simulink model "Vector_projection_get_closest_point"  (R2021a)
settings: configuration reference "AION_IDS_Speedgoat" (kept outside this file)
libraries: simulink x1
Description:
  | 向量投影法获取线段P1P2上距离当前点P的最近点C
settings Model: DataDictionary=Vector_Projection_Get_Closest_Point.sldd  Creator=xinrui  LastModifiedBy=Administrator
settings ConfigSetRef: SourceName=AION_IDS_Speedgoat

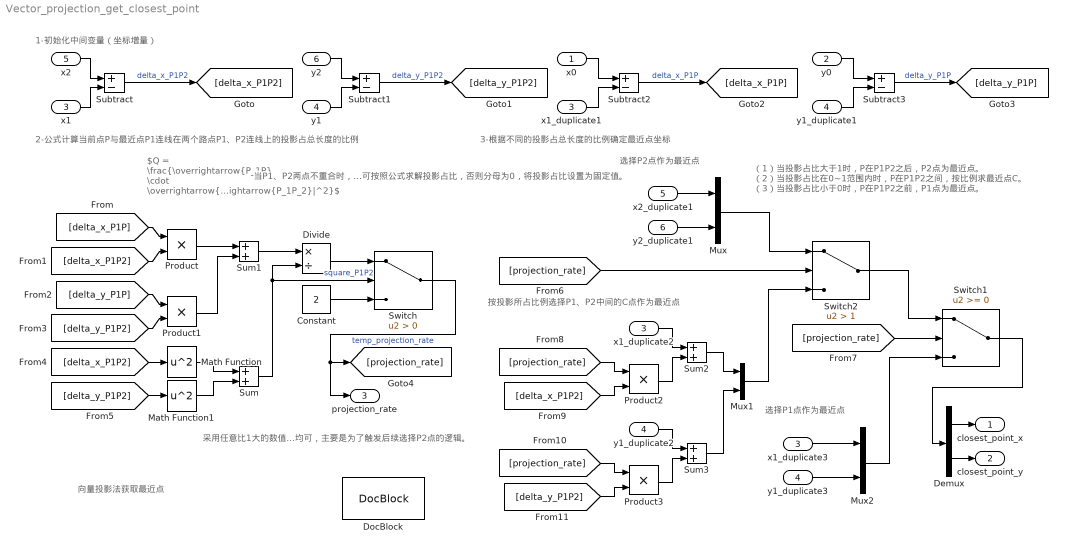
== system Vector_projection_get_closest_point ==
  note: $Q = \frac{\overrightarrow{P_1P} \cdot \overrightarrow{P_1P_2}}{|\overrightarrow{P_1P_2}|^2}$
  note: 当P1、P2两点不重合时，可按照公式求解投影占比，否则分母为0，将投影占比设置为固定值。
  note: （1）当投影占比大于1时，P在P1P2之后，P2点为最近点。
      | （2）当投影占比在0~1范围内时，P在P1P2之间，按比例求最近点C。
      | （3）当投影占比小于0时，P在P1P2之前，P1点为最近点。
  note: 向量投影法获取最近点
  note: 选择P1点作为最近点
  note: 按投影所占比例选择P1、P2中间的C点作为最近点
  note: 选择P2点作为最近点
  note: 采用任意比1大的数值均可，主要是为了触发后续选择P2点的逻辑。
  note: 3-根据不同的投影占总长度的比例确定最近点坐标
  note: 2-公式计算当前点P与最近点P1连线在两个路点P1、P2连线上的投影占总长度的比例
  note: 1-初始化中间变量（坐标增量）
  x0 : Inport  Description=当前点P的x坐标，实数，m。  OutDataTypeStr=double  PortDimensions=1
  y0 : Inport  Description=当前点P的y坐标，实数，m。  Port=2  OutDataTypeStr=double  PortDimensions=1
  x1 : Inport  Description=路点线段起始端点P1的x坐标，实数，m。  Port=3  OutDataTypeStr=double  PortDimensions=1
  y1 : Inport  Description=路点线段起始端点P1的y坐标，实数，m。  Port=4  OutDataTypeStr=double  PortDimensions=1
  x2 : Inport  Description=路点线段终止端点P2的x坐标，实数，m。  Port=5  OutDataTypeStr=double  PortDimensions=1
  y2 : Inport  Description=路点线段终止端点P2的y坐标，实数，m。  Port=6  OutDataTypeStr=double  PortDimensions=1
  Constant : Constant  Description=采用任意比1大的数值均可，主要是为了触发后续选择P2点的逻辑。  Value=2  OutDataTypeStr=double
  Demux : Demux  Outputs=2
  Divide : Product  Description=公式计算当前点P与最近点P1连线在两个路点P1、P2连线上的投影占总长度的比例  Inputs=*/
  DocBlock : simulink/Model-Wide Utilities/DocBlock  DocumentType=HTML  mask(DocBlock){}
      mask Display:
      | plot([.8 0 0 1 1 .8 .8 1],[1 1 0 0 .8 1 .8 .8]);
      | text(.5,.6,'CHANGELOG','horizontalalignment','center');
      | text(.95,.05,get_param(gcb,'DocumentType'),'verticalalignment','bottom','horizontalalignment','right');
  Math Function : Math  Operator=square  SaturateOnIntegerOverflow=on
  Math Function1 : Math  Operator=square  SaturateOnIntegerOverflow=on
  Mux : Mux  Inputs=2
  Mux1 : Mux  Inputs=2
  Mux2 : Mux  Inputs=2
  Product{,1..3} (4 alike) : Product
  Subtract : Sum  Description=计算线段P1P2的x坐标增量。  Inputs=+-
  Subtract1 : Sum  Description=计算线段P1P2的y坐标增量。  Inputs=+-
  Subtract2 : Sum  Description=计算线段P1P的x坐标增量。  Inputs=+-
  Subtract3 : Sum  Description=计算线段P1P的y坐标增量。  Inputs=+-
  Sum : Sum  Description=计算线段P1P2的距离平方，以判断公式分母是否为零。
  Sum1 : Sum
  Sum2 : Sum  Description=按投影所占比例选择P1、P2中间的C点作为最近点。
  Sum3 : Sum  Description=按投影所占比例选择P1、P2中间的C点作为最近点。
  Switch : Switch  Description=当P1、P2两点不重合时，可按照公式求解投影占比，否则分母为0，将投影占比设置为固定值。  Criteria=u2 > Threshold  OutDataTypeStr=double
  Switch1 : Switch  Description=|  OutDataTypeStr=double
      | （1）当投影占比大于1时，P在P1P2之后，P2点为最近点。
      | （2）当投影占比在0~1范围内时，P在P1P2之间，按比例求最近点C。
      | （3）当投影占比小于0时，P在P1P2之前，P1点为最近点。
  Switch2 : Switch  Description=|  Criteria=u2 > Threshold  Threshold=1  OutDataTypeStr=double
      | （1）当投影占比大于1时，P在P1P2之后，P2点为最近点。
      | （2）当投影占比在0~1范围内时，P在P1P2之间，按比例求最近点C。
      | （3）当投影占比小于0时，P在P1P2之前，P1点为最近点。
  x1_duplicate1 : InportShadow  Port=3  OutDataTypeStr=double  PortDimensions=1
  x1_duplicate2 : InportShadow  Port=3  OutDataTypeStr=double  PortDimensions=1
  x1_duplicate3 : InportShadow  Port=3  OutDataTypeStr=double  PortDimensions=1
  x2_duplicate1 : InportShadow  Port=5  OutDataTypeStr=double  PortDimensions=1
  y1_duplicate1 : InportShadow  Port=4  OutDataTypeStr=double  PortDimensions=1
  y1_duplicate2 : InportShadow  Port=4  OutDataTypeStr=double  PortDimensions=1
  y1_duplicate3 : InportShadow  Port=4  OutDataTypeStr=double  PortDimensions=1
  y2_duplicate1 : InportShadow  Port=6  OutDataTypeStr=double  PortDimensions=1
  closest_point_x : Outport  Description=路点线段上距离当前点P最近的点C的x坐标，实数，m。  OutDataTypeStr=double  PortDimensions=1
  closest_point_y : Outport  Description=路点线段上距离当前点P最近的点C的y坐标，实数，m。  Port=2  OutDataTypeStr=double  PortDimensions=1
  projection_rate : Outport  Description=当前点P与线段起始点P1连线在两个路点P1、P2连线上的投影占总长度的比例，实数，无量纲。  Port=3  OutDataTypeStr=double  PortDimensions=1
  wires:
  x0/1 -> Subtract2/1
  x2/1 -> Subtract/1
  x1/1 -> Subtract/2
  y2/1 -> Subtract1/1
  y1/1 -> Subtract1/2
  y0/1 -> Subtract3/1
  Math Function/1 -> Sum/1
  Math Function1/1 -> Sum/2
  Sum/1 -> Divide/2, Switch/2  "square_P1P2"
  Product/1 -> Sum1/1
  Product1/1 -> Sum1/2
  Sum1/1 -> Divide/1
  Divide/1 -> Switch/1
  Constant/1 -> Switch/3
  Mux/1 -> Switch2/1
  Product2/1 -> Sum2/2
  Product3/1 -> Sum3/2
  Sum2/1 -> Mux1/1
  Sum3/1 -> Mux1/2
  Mux1/1 -> Switch2/3
  Switch2/1 -> Switch1/1
  Mux2/1 -> Switch1/3
  Switch1/1 -> Demux/1
  Demux/1 -> closest_point_x/1
  Demux/2 -> closest_point_y/1
  Subtract/1 -> [delta_x_P1P2]  "delta_x_P1P2"
  Subtract1/1 -> [delta_y_P1P2]  "delta_y_P1P2"
  x1_duplicate1/1 -> Subtract2/2
  Subtract2/1 -> [delta_x_P1P]  "delta_x_P1P"
  y1_duplicate1/1 -> Subtract3/2
  Subtract3/1 -> [delta_y_P1P]  "delta_y_P1P"
  [delta_x_P1P] -> Product/1
  [delta_x_P1P2] -> Product/2
  [delta_y_P1P] -> Product1/1
  [delta_y_P1P2] -> Product1/2
  [delta_y_P1P2] -> Math Function1/1
  [delta_x_P1P2] -> Math Function/1
  Switch/1 -> [projection_rate], projection_rate/1  "temp_projection_rate"
  [projection_rate] -> Switch2/2
  [projection_rate] -> Switch1/2
  x2_duplicate1/1 -> Mux/1
  y2_duplicate1/1 -> Mux/2
  x1_duplicate2/1 -> Sum2/1
  [projection_rate] -> Product2/1
  [delta_x_P1P2] -> Product2/2
  y1_duplicate2/1 -> Sum3/1
  [projection_rate] -> Product3/1
  [delta_y_P1P2] -> Product3/2
  x1_duplicate3/1 -> Mux2/1
  y1_duplicate3/1 -> Mux2/2
